simulink model "PreisachSimulation"  (R2017b)
settings: Solver=VariableStepAuto  StartTime=0.0  StopTime=simTotalTime  FixedStep=0.05  MaxStep=0.1  MinStep=0.01  RelTol=1e-3
undefined symbols (not defined in the file): initialInput, inputMax, inputMin, outputMax, outputMin, simTotalTime
libraries: simulink x1
settings Model: Creator=Marco  LastModifiedBy=M. Vasquez Beltran

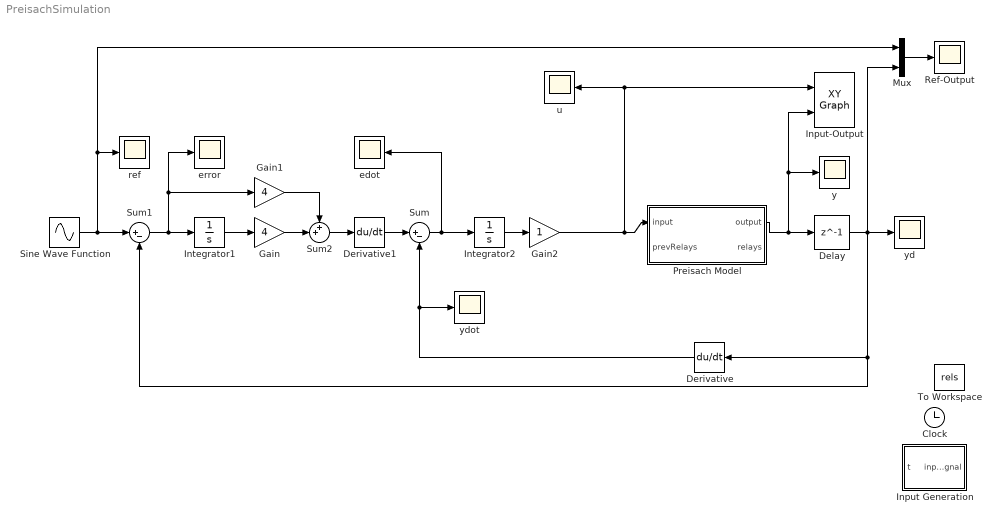
== system PreisachSimulation ==
  Clock : Clock
  Delay : Delay  DelayLength=1
  Derivative : Derivative  CoefficientInTFapproximation=100
  Derivative1 : Derivative
  Gain : Gain  Gain=4
  Gain1 : Gain  Gain=4
  Gain2 : Gain
  Input Generation : MATLAB Function  TreatAsAtomicUnit=on
  Input-Output : simulink/Sinks/XY Graph  xmin=inputMin*1.25  xmax=inputMax*1.25  ymin=outputMin*1.25  ymax=outputMax*1.25  st=-1
  Integrator1 : Integrator
  Integrator2 : Integrator
  Mux : Mux  Inputs=2
  Preisach Model : MATLAB Function  TreatAsAtomicUnit=on
  Ref-Output : Scope
  Sine Wave Function : Sin  Amplitude=100  Bias=200  Frequency=2*pi/50  SampleTime=0
  Sum : Sum  Inputs=|+-
  Sum1 : Sum  Inputs=|+-
  Sum2 : Sum  Inputs=++|
  To Workspace : ToWorkspace  VariableName=rels  SampleTime=-1
  edot : Scope
  error : Scope
  ref : Scope
  u : Scope
  y : Scope
  yd : Scope
  ydot : Scope
  wires:
  Derivative1/1 -> Sum/1
  Sum/1 -> Integrator2/1, edot/1
  Sum1/1 -> Gain1/1, error/1, Integrator1/1
  Integrator1/1 -> Gain/1
  Gain/1 -> Sum2/2
  Gain1/1 -> Sum2/1
  Sine Wave Function/1 -> Sum1/1, Mux/1, ref/1
  Sum2/1 -> Derivative1/1
  Mux/1 -> Ref-Output/1
  Integrator2/1 -> Gain2/1
  Derivative/1 -> ydot/1, Sum/2
  Preisach Model/1(output) -> Delay/1, Input-Output/2, y/1
  Gain2/1 -> Input-Output/1, u/1, Preisach Model/1(input)
  Delay/1 -> yd/1, Sum1/2, Derivative/1, Mux/2

== matlab function PreisachSimulation/Input Generation ==
  data: t input; simTotalTime parameter; inputSignal output; inputMin parameter; inputMax parameter; initialInput parameter
function inputSignal = fcn(t,...
    simTotalTime, inputMin, inputMax, initialInput)

timeDecreasingFactor = ( simTotalTime - 0.3*t )/simTotalTime;

inputMinFactor = 1.00;
inputMaxFactor = 1.00;

amplitude = (inputMaxFactor*inputMax - inputMinFactor*inputMin)/2;
% amplitude = timeDecreasingFactor*(inputMaxFactor*inputMax - inputMinFactor*inputMin)/2;
offset = (inputMaxFactor*inputMax + inputMinFactor*inputMin)/2;
freq = 1/40;
phase = -asin((initialInput - offset)/amplitude);

% amplitude = 3;
% offset = -3;
% freq = 1/40;
% phase = 0;

inputSignal = amplitude * sin( 2*pi*freq*t - phase ) + offset;

== matlab function PreisachSimulation/Preisach Model ==
  data: input input; prevRelays input; output output; preisachRelayModel parameter; relays output
function [output, relays] = fcn(input, prevRelays, ...
    preisachRelayModel)

% prevRelays, n, alphabeta, mu, disArea, hysteronMin, hysteronMax, shift
output=shift;
relays=prevRelays;
for i=1:n
    ii = n-i+1;
    for j=1:i
        if( input <= alphabeta(j) ) 
            relays(ii,j) = hysteronMin; 
        elseif( input >= alphabeta(i) ) 
            relays(ii,j) = hysteronMax;
        end
        output = output + relays(ii,j)*mu(ii,j)*disArea;
        output = output + relays(ii,j)*mu(ii,j);
    end
end
